simulink model "Test_model"  (R2020b)
settings: Solver=VariableStepAuto  StartTime=0.0  StopTime=500  RelTol=1e-3
undefined symbols (not defined in the file or in its folder): Alin, Blin, Clin, Dlin
libraries: pid_lib x2, rllib x1, powerlib_meascontrol x1
settings Model: PacingRate=0.100000  Creator=Xiong  LastModifiedBy=Xiong
settings DataIOCC: ExternalInput=getinputstruct(report1)  InitialState=getstatestruct(report1)

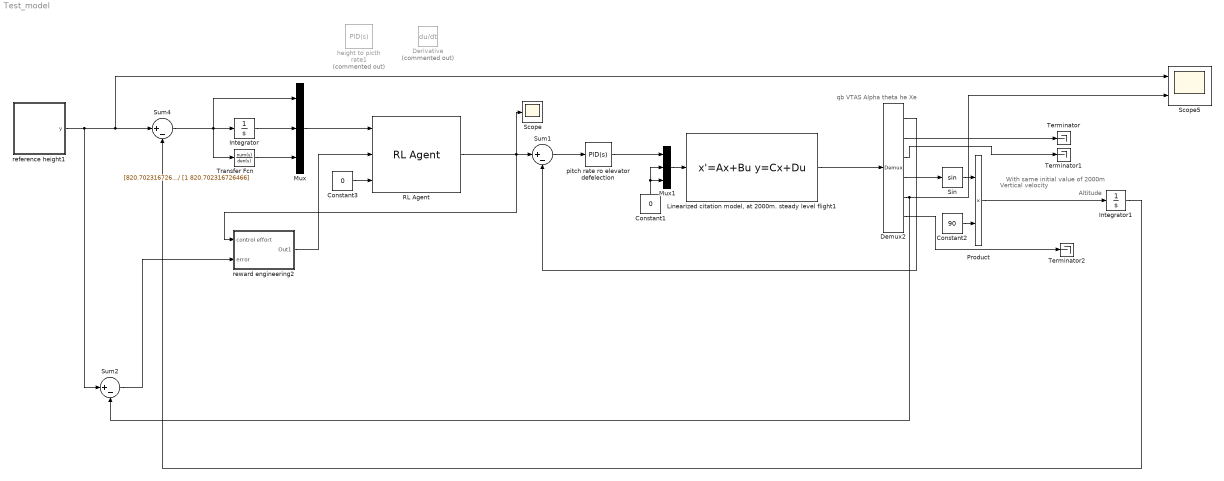
== system Test_model ==
  note: Vertical velocity
  note: With same initial value of 2000m
  note: Altitude
  note: qb
      |
      | VTAS
      |
      | Alpha
      |
      | theta
      |
      | he
      |
      | Xe
  Constant1 : Constant  Value=0
  Constant2 : Constant  Value=90
  Constant3 : Constant  Value=0
  Demux2 : Demux  Outputs=6
  Derivative : Derivative  Commented=on
  Integrator : Integrator
  Integrator1 : Integrator
  "Linearized citation model, at 2000m. steady level flight1" : StateSpace  A=Alin  B=Blin  C=Clin  D=Dlin  InitialCondition=0
      mask Display: image('C:\Program Files\MATLAB\R2020b\Jiajiadebiyesheji\Citation simulation model\Citation.jpg'); % Use "Edit Image" on toolstrip to change.
  Mux : Mux  Inputs=3
  Mux1 : Mux  Inputs=3
  Product : Product
  RL Agent : rllib/RL Agent  Agent=agent  ProvideReward=on  ProvideIsDone=on  ProvideCumRwd=off  TreatAsDirectFeedthrough=on  CollectLoggedSignals=on  CollectModelStates=on
  Scope : Scope
  Scope5 : Scope  NumInputPorts=2
  Sin : Trigonometry
  Sum1 : Sum  Inputs=|+-
  Sum2 : Sum  Inputs=|+-
  Sum4 : Sum  Inputs=|+-
  Terminator : Terminator
  Terminator1 : Terminator
  Terminator2 : Terminator
  Transfer Fcn : TransferFcn  Numerator=[820.702316726466 0]  Denominator=[1 820.702316726466]
  height to picth rate1 : pid_lib/PID Controller  Commented=on  Controller=PID  Form=Parallel  TimeDomain=Continuous-time  UseExternalTs=off  SampleTime=-1  IntegratorMethod=Forward Euler  FilterMethod=Forward Euler  ControllerParametersSource=internal  P=0.0136796702122434  I=0.000573114709441426  D=0.0725488731732448  UseFilter=on  N=820.702316726466  TunerSelectOption=Transfer Function Based (PID Tuner App)  InitialConditionSource=internal  InitialConditionForIntegrator=0  InitialConditionForFilter=0  DifferentiatorICPrevScaledInput=0  ExternalReset=none  TrackingMode=off  Kt=1  LimitOutput=off  SatLimitsSource=internal  UpperSaturationLimit=inf  LowerSaturationLimit=-inf  LinearizeAsGain=on  AntiWindupMode=none  Kb=1  POutMin=[]  POutMax=[]  IOutMin=[]  IOutMax=[]  DOutMin=[]  DOutMax=[]  NOutMin=[]  NOutMax=[]  SumOutMin=[]  SumOutMax=[]  SaturationOutMin=[]  SaturationOutMax=[]  PParamMin=[]  PParamMax=[]  IParamMin=[]  IParamMax=[]  DParamMin=[]  DParamMax=[]  NParamMin=[]  NParamMax=[]  KbParamMin=[]  KbParamMax=[]  KtParamMin=[]  KtParamMax=[]  KbOutMin=[]  KbOutMax=[]  KtOutMin=[]  KtOutMax=[]  IntegratorOutMin=[]  IntegratorOutMax=[]  FilterOutMin=[]  FilterOutMax=[]  SumI1OutMin=[]  SumI1OutMax=[]  SumI2OutMin=[]  SumI2OutMax=[]  SumI3OutMin=[]  SumI3OutMax=[]  SumI4OutMin=[]  SumI4OutMax=[]  SumDOutMin=[]  SumDOutMax=[]  DifferentiatorOutMin=[]  DifferentiatorOutMax=[]  FilterDiffOutCoefMin=[]  FilterDiffOutCoefMax=[]  ReciprocalOutMin=[]  ReciprocalOutMax=[]  SumDenOutMin=[]  SumDenOutMax=[]  SumNumOutMin=[]  SumNumOutMax=[]  DivideOutMin=[]  DivideOutMax=[]  UdiffTsProdOutMin=[]  UdiffTsProdOutMax=[]  NTsProdOutMin=[]  NTsProdOutMax=[]  UintegralTsProdOutMin=[]  UintegralTsProdOutMax=[]  UngainTsProdOutMin=[]  UngainTsProdOutMax=[]  IntegratorContinuousStateAttributes=''  IntegratorStateMustResolveToSignalObject=off  IntegratorRTWStateStorageClass=Auto  FilterContinuousStateAttributes=''  FilterStateMustResolveToSignalObject=off  FilterRTWStateStorageClass=Auto  ParallelPVariant=InternalParameters  IdealPVariant=Disabled  IVariant=InternalParameters  DVariant=InternalParameters  IntegratorVariant=Continuous  SatVariant=Disabled  AWVariant=Passthrough  PCopyVariant=Disabled  TRVariant=Disabled  FdbkBlocksVariant=Forward  IdealPFdbkVariant=Disabled  SatFdbkVariant=Disabled  DerivativeFilterVariant=ContFilter  NVariant=InternalParameters  NCopyVariant=Disabled  FilterICVariant=InternalICsFilter  IntegratorICVariant=InternalICs  ExternalResetVariant=Disabled  TRSumVariant=Passthrough  SumFdbkVariant=Disabled  SumVariant=Sum_PID  TsampFilterVariant=InternalTs  TsampNgainVariant=Passthrough  TsampIntegralVariant=Passthrough  ExternalSaturationOutDataTypeStr=Inherit: Same as second input
  pitch rate ro elevator defelection : pid_lib/PID Controller  Controller=PID  Form=Parallel  TimeDomain=Continuous-time  UseExternalTs=off  SampleTime=-1  IntegratorMethod=Forward Euler  FilterMethod=Forward Euler  ControllerParametersSource=internal  P=-1.62745526673808  I=-18.745171116188  D=-0.0318627725221163  UseFilter=on  N=229.233229472629  TunerSelectOption=Transfer Function Based (PID Tuner App)  InitialConditionSource=internal  InitialConditionForIntegrator=0  InitialConditionForFilter=0  DifferentiatorICPrevScaledInput=0  ExternalReset=none  TrackingMode=off  Kt=1  LimitOutput=off  SatLimitsSource=internal  UpperSaturationLimit=inf  LowerSaturationLimit=-inf  LinearizeAsGain=on  AntiWindupMode=none  Kb=1  POutMin=[]  POutMax=[]  IOutMin=[]  IOutMax=[]  DOutMin=[]  DOutMax=[]  NOutMin=[]  NOutMax=[]  SumOutMin=[]  SumOutMax=[]  SaturationOutMin=[]  SaturationOutMax=[]  PParamMin=[]  PParamMax=[]  IParamMin=[]  IParamMax=[]  DParamMin=[]  DParamMax=[]  NParamMin=[]  NParamMax=[]  KbParamMin=[]  KbParamMax=[]  KtParamMin=[]  KtParamMax=[]  KbOutMin=[]  KbOutMax=[]  KtOutMin=[]  KtOutMax=[]  IntegratorOutMin=[]  IntegratorOutMax=[]  FilterOutMin=[]  FilterOutMax=[]  SumI1OutMin=[]  SumI1OutMax=[]  SumI2OutMin=[]  SumI2OutMax=[]  SumI3OutMin=[]  SumI3OutMax=[]  SumI4OutMin=[]  SumI4OutMax=[]  SumDOutMin=[]  SumDOutMax=[]  DifferentiatorOutMin=[]  DifferentiatorOutMax=[]  FilterDiffOutCoefMin=[]  FilterDiffOutCoefMax=[]  ReciprocalOutMin=[]  ReciprocalOutMax=[]  SumDenOutMin=[]  SumDenOutMax=[]  SumNumOutMin=[]  SumNumOutMax=[]  DivideOutMin=[]  DivideOutMax=[]  UdiffTsProdOutMin=[]  UdiffTsProdOutMax=[]  NTsProdOutMin=[]  NTsProdOutMax=[]  UintegralTsProdOutMin=[]  UintegralTsProdOutMax=[]  UngainTsProdOutMin=[]  UngainTsProdOutMax=[]  IntegratorContinuousStateAttributes=''  IntegratorStateMustResolveToSignalObject=off  IntegratorRTWStateStorageClass=Auto  FilterContinuousStateAttributes=''  FilterStateMustResolveToSignalObject=off  FilterRTWStateStorageClass=Auto  ParallelPVariant=InternalParameters  IdealPVariant=Disabled  IVariant=InternalParameters  DVariant=InternalParameters  IntegratorVariant=Continuous  SatVariant=Disabled  AWVariant=Passthrough  PCopyVariant=Disabled  TRVariant=Disabled  FdbkBlocksVariant=Forward  IdealPFdbkVariant=Disabled  SatFdbkVariant=Disabled  DerivativeFilterVariant=ContFilter  NVariant=InternalParameters  NCopyVariant=Disabled  FilterICVariant=InternalICsFilter  IntegratorICVariant=InternalICs  ExternalResetVariant=Disabled  TRSumVariant=Passthrough  SumFdbkVariant=Disabled  SumVariant=Sum_PID  TsampFilterVariant=InternalTs  TsampNgainVariant=Passthrough  TsampIntegralVariant=Passthrough  ExternalSaturationOutDataTypeStr=Inherit: Same as second input
  reference height1 : Subsystem
  reward engineering2 : Subsystem
  wires:
  Demux2/1 -> Sum1/2
  Demux2/4 -> Sin/1
  Integrator/1 -> Mux/2
  Constant1/1 -> Mux1/2, Mux1/3
  Transfer Fcn/1 -> Mux/3
  Sum4/1 -> Transfer Fcn/1, Mux/1, Integrator/1
  Sum1/1 -> pitch rate ro elevator defelection/1
  reference height1/1(y) -> Scope5/1, Sum4/1, Sum2/1
  Sum2/1 -> reward engineering2/2(error)
  "Linearized citation model, at 2000m. steady level flight1"/1 -> Demux2/1
  pitch rate ro elevator defelection/1 -> Mux1/1
  Integrator1/1 -> Sum4/2
  Sin/1 -> Product/1
  Demux2/3 -> Terminator1/1
  RL Agent/1 -> Sum1/1, Scope/1, reward engineering2/1(control effort)
  Demux2/5 -> Scope5/2, Sum2/2
  reward engineering2/1(Out1) -> RL Agent/2
  Demux2/2 -> Terminator/1
  Mux1/1 -> "Linearized citation model, at 2000m. steady level flight1"/1
  Constant2/1 -> Product/2
  Demux2/6 -> Terminator2/1
  Product/1 -> Integrator1/1
  Constant3/1 -> RL Agent/3
  Mux/1 -> RL Agent/1

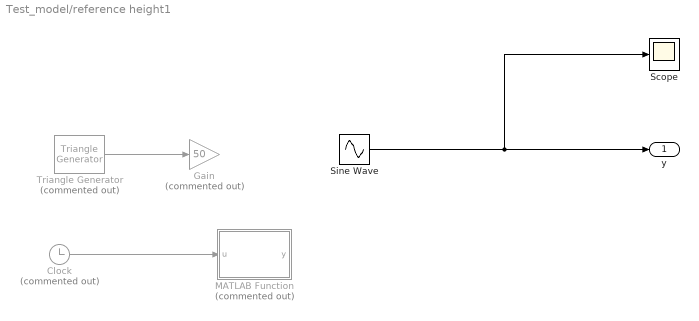
== system Test_model/reference height1 ==
  Clock : Clock  Commented=on
  Gain : Gain  Commented=on  Gain=50
  MATLAB Function : MATLAB Function  Commented=on  TreatAsAtomicUnit=on
  Scope : Scope
  Sine Wave : Sin  Amplitude=50  Frequency=2*pi/20  SampleTime=0
  Triangle Generator : powerlib_meascontrol/Pulse & Signal Generators/Triangle Generator  Commented=on  Freq=0.025  Phase=90  Ts=0
  y : Outport
  wires:
  Clock/1 -> MATLAB Function/1(u)
  Triangle Generator/1 -> Gain/1
  Sine Wave/1 -> Scope/1, y/1

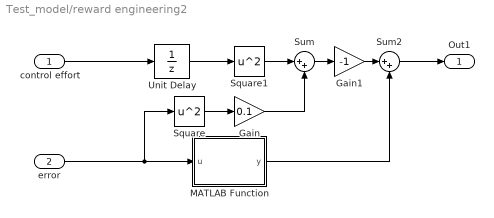
== system Test_model/reward engineering2 ==
  control effort : Inport
  error : Inport  Port=2
  Gain : Gain  Gain=0.1
  Gain1 : Gain  Gain=-1
  MATLAB Function : MATLAB Function  TreatAsAtomicUnit=on
  Square : Math  Operator=square  SaturateOnIntegerOverflow=on
  Square1 : Math  Operator=square  SaturateOnIntegerOverflow=on
  Sum : Sum  Inputs=|++
  Sum2 : Sum  Inputs=|++
  Unit Delay : UnitDelay  SampleTime=-1  HasFrameUpgradeWarning=on
  Out1 : Outport
  wires:
  MATLAB Function/1(y) -> Sum2/2
  Unit Delay/1 -> Square1/1
  Square/1 -> Gain/1
  Gain1/1 -> Sum2/1
  Gain/1 -> Sum/2
  Sum/1 -> Gain1/1
  error/1 -> Square/1, MATLAB Function/1(u)
  control effort/1 -> Unit Delay/1
  Square1/1 -> Sum/1
  Sum2/1 -> Out1/1

== matlab function Test_model/reward engineering2/MATLAB Function ==
  data: u input; y output
function y = fcn(u)
if u^2<69
    y=1
else
    y=0
end

== matlab function Test_model/reference height1/MATLAB Function ==
  data: u input; y output
function y = fcn(u)
if u < 8
    y = 0
elseif u>8 & u <12
    y = -80+10*u
elseif u >=12
    y = 40
else
    y = 0
end
